simulink model "ContainerVesselDDPG"  (R2022a)
settings: Solver=ode3  StartTime=0.0  StopTime=600.0  FixedStep=0.1  RelTol=1e-3  EnableMultiTasking=on
libraries: simulink x2, rllib x1
settings Model: Creator=hntran  LastModifiedBy=hntran
settings SolverCC: AlgebraicLoopSolver=TrustRegion
settings DataIOCC: LimitDataPoints=on  SaveFormat=Array  SignalLoggingSaveFormat=ModelDataLogs  ReturnWorkspaceOutputs=off
settings OptimizationCC: InitFltsAndDblsToZero=on  LifeSpan=inf
settings DebuggingCC: SaveWithParameterizedLinksMsg=none  UnderspecifiedInitializationDetection=Classic  MergeDetectMultiDrivingBlocksExec=none  SignalResolutionControl=TryResolveAllWithWarning  SolverPrmCheckMsg=warning  MultiTaskDSMMsg=warning  MultiTaskCondExecSysMsg=none  FcnCallInpInsideContextMsg=warning  UnconnectedInputMsg=warning  UnconnectedOutputMsg=warning  UnconnectedLineMsg=warning  SFUnexpectedBacktrackingDiag=warning  SFNoUnconditionalDefaultTransitionDiag=warning  SFExecutionAtInitializationDiag=none  SFMachineParentedDataDiag=warning  ArithmeticOperatorsInVariantConditions=warning
settings HardwareCC: ProdBitPerPointer=32  ProdBitPerSizeT=32  ProdBitPerPtrDiffT=32  ProdLargestAtomicFloat=None  ProdIntDivRoundTo=Undefined  ProdEndianess=Unspecified  ProdWordSize=32  ProdHWDeviceType=32-bit Generic
settings ModelReferenceCC: PropagateSignalLabelsOutOfModel=off
settings CodeAppCC: StateflowObjectComments=on
settings GRTTargetCC: TargetFcnLib=ansi_tfl_tmw.mat  TargetLangStandard=C89/C90 (ANSI)  CombineOutputUpdateFcns=off  GRTInterface=on
settings ConfigComp: CovMetricSettings=dw  CovSaveCumulativeToWorkspaceVar=on  CovSaveSingleToWorkspaceVar=on

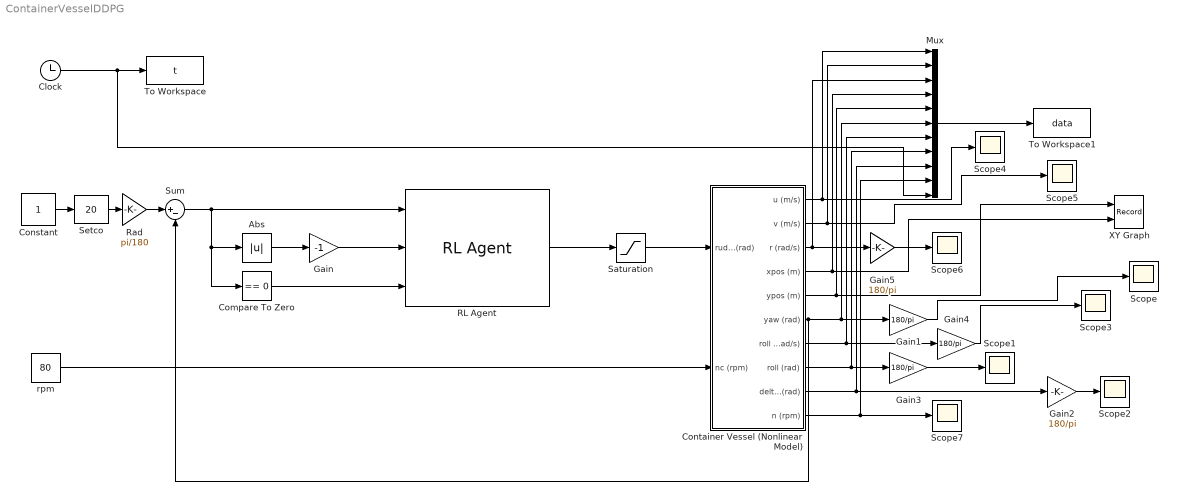
== system ContainerVesselDDPG ==
  Abs : Abs  SaturateOnIntegerOverflow=off
  Clock : Clock
  Compare To Zero : simulink/Logic and Bit Operations/Compare To Zero  relop===  OutDataTypeStr=boolean
  Constant : Constant
  Container Vessel (Nonlinear Model) : Subsystem
  Gain : Gain  Gain=-1
  Gain{1..5} (5 alike) : Gain  Gain=180/pi
  Mux : Mux  Inputs=11
  RL Agent : rllib/RL Agent  Agent=agent  ExternalActionAsInput=off  ProvideLastAction=off  ProvideCumRwd=off  TreatAsDirectFeedthrough=on  UseStrictObservationDataTypes=off
  Rad : Gain  Gain=pi/180  SaturateOnIntegerOverflow=on  OutDataTypeStr=Inherit: Same as input  ParamDataTypeStr=Inherit: Same as input
  Saturation : Saturate  UpperLimit=10*pi/180  LowerLimit=-10*pi/180
  Scope{,1..7} (8 alike) : Scope
  Setco : simulink/Math Operations/Slider Gain  gain=20  low=0  high=360
  Sum : Sum  Inputs=|+-
  To Workspace : ToWorkspace  VariableName=t  SampleTime=-1
  To Workspace1 : ToWorkspace  VariableName=data  SampleTime=-1
      settings: Decimation=2
  XY Graph : Record  FileSettingsInternal="{\"entries\":[{\"content\":{\"excelSettings\":{\"content\":{},\"type\":\"Streamout.ExcelSettings\"}},\"type\":\"Streamout.FileSettingStorage\",\"uuid\":\"f43c24fc-feab-4f1a-8c9e-b8f5f69fa37c\"}],\"packageUris\":[\"http://schema.mathworks.com/mf0/streamout_blocks/R2020a\"],\"version\":\"1.0\"}"  Layout=[1 1]  SignalsInternal="{\"entries\":[{\"content\":{\"signals\":[{\"content\":{\"blockPath\":[\"ContainerVesselDDPG/XY Graph\"],\"channel\":[],\"dimensions\":[1],\"domain\":\"ContainerVesselDDPG/XY Graph\",\"lineColor\":\"#a2142f\",\"plots\":[1],\"port\":1,\"sid\":[],\"signalID\":3378,\"signalName\":\"XY Graph:1\"},\"type\":\"RecordBlkView.Signal\",\"uuid\":\"135c65cd-a5f0-4a3b-81cf-bed84d498486\"},{\"content\":{\"blockPath\":[\"ContainerVesselDDPG/XY Graph\"],\"channel\":[],\"dimensions\":[1],\"domain\":\"ContainerVesselDDPG/XY Graph\",\"lineColor\":\"#139fff\",\"plots\":[1],\"port\":2,\"sid\":[],\"signalID\":3381,\"signalName\":\"XY Graph:2\"},\"type\":\"RecordBlkView.Signal\",\"uuid\":\"91a8dce2-58e7-4733-aea4-42f3c8218d35\"}]},\"type\":\"RecordBlkView.InputSignals\",\"uuid\":\"c6774691-92ed-4fab-83e8-d291ec8d1e7a\"}],\"packageUris\":[\"http://schema.mathworks.com/mf0/streamout_blocks/R2020a\"],\"version\":\"1.0\"}"  VisualizationBindings="{\"xyplotplugin\":{\"info\":[{\"series\":[{\"bindingParametersList\":[{\"parameter\":\"X-Axis\",\"signalID\":3378,\"signalName\":\"XY Graph:1\"},{\"parameter\":\"Y-Axis\",\"signalID\":3381,\"signalName\":\"XY Graph:2\"}],\"seriesID\":48504}],\"subplotID\":1}]}}"  CompatibilityTag=XY  st=-1
  rpm : Constant  Value=80
  wires:
  Clock/1 -> To Workspace/1, Mux/11
  rpm/1 -> Container Vessel (Nonlinear Model)/2(nc (rpm))
  Container Vessel (Nonlinear Model)/4(xpos (m)) -> XY Graph/2, Mux/4
  Container Vessel (Nonlinear Model)/5(ypos (m)) -> XY Graph/1, Mux/5
  Container Vessel (Nonlinear Model)/6(yaw (rad)) -> Gain1/1, Mux/6, Sum/2
  Gain1/1 -> Scope/1
  Container Vessel (Nonlinear Model)/9(delta (rad)) -> Gain2/1, Mux/9
  Gain2/1 -> Scope2/1
  Container Vessel (Nonlinear Model)/8(roll (rad)) -> Gain3/1, Mux/8
  Gain3/1 -> Scope1/1
  Container Vessel (Nonlinear Model)/7(roll rate (rad/s)) -> Gain4/1, Mux/7
  Gain4/1 -> Scope3/1
  Mux/1 -> To Workspace1/1
  Container Vessel (Nonlinear Model)/1(u (m/s)) -> Scope4/1, Mux/1
  Container Vessel (Nonlinear Model)/2(v (m/s)) -> Scope5/1, Mux/2
  Container Vessel (Nonlinear Model)/3(r (rad/s)) -> Gain5/1, Mux/3
  Gain5/1 -> Scope6/1
  Container Vessel (Nonlinear Model)/10(n (rpm)) -> Scope7/1, Mux/10
  Constant/1 -> Setco/1
  Setco/1 -> Rad/1
  Saturation/1 -> Container Vessel (Nonlinear Model)/1(rudc (rad))
  Rad/1 -> Sum/1
  RL Agent/1 -> Saturation/1
  Sum/1 -> Compare To Zero/1, Abs/1, RL Agent/1
  Abs/1 -> Gain/1
  Gain/1 -> RL Agent/2
  Compare To Zero/1 -> RL Agent/3

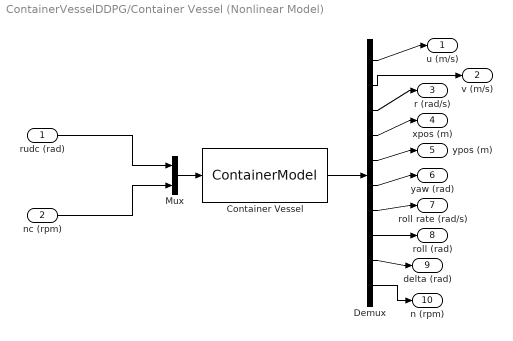
== system ContainerVesselDDPG/Container Vessel (Nonlinear Model) ==
  rudc (rad) : Inport
  nc (rpm) : Inport  Port=2
  Container Vessel : S-Function  FunctionName=ContainerModel  SFunctionDeploymentMode=off  EnableBusSupport=off
  Demux : Demux  Outputs=10
  Mux : Mux  Inputs=2
  u (m/s) : Outport
  v (m/s) : Outport  Port=2
  r (rad/s) : Outport  Port=3
  xpos (m) : Outport  Port=4
  ypos (m) : Outport  Port=5
  yaw (rad) : Outport  Port=6
  roll rate (rad/s) : Outport  Port=7
  roll (rad) : Outport  Port=8
  delta (rad) : Outport  Port=9
  n (rpm) : Outport  Port=10
  wires:
  Mux/1 -> Container Vessel/1
  Container Vessel/1 -> Demux/1
  Demux/1 -> u (m/s)/1
  Demux/2 -> v (m/s)/1
  Demux/3 -> r (rad/s)/1
  Demux/4 -> xpos (m)/1
  Demux/5 -> ypos (m)/1
  Demux/6 -> yaw (rad)/1
  nc (rpm)/1 -> Mux/2
  Demux/7 -> roll rate (rad/s)/1
  Demux/8 -> roll (rad)/1
  Demux/9 -> delta (rad)/1
  Demux/10 -> n (rpm)/1
  rudc (rad)/1 -> Mux/1
